simulink model "tpi_sim"  (R2019a)
settings: Solver=VariableStepDiscrete  StartTime=0.0  StopTime=inf  RelTol=1e-3
values from neighbouring files (symbols this model uses):
  tbd1 = 5*(stages1 - 1)    (= 30)    [simloop_and_plot.m]
  tbd2 = 5*(stages2 - 1)    (= 10)    [simloop_and_plot.m]
  tbd3 = 5*(stages3 - 1)    (= 20)    [simloop_and_plot.m]
  tbd4 = 5*(stages4 - 1)    (= 40)    [simloop_and_plot.m]
libraries: commdigbbndpm3 x18, commcnvcod2 x18, commchan3 x14, commutil2 x14, commsink2 x14, commrandsrc3 x14, commdigbbndam3 x8
settings Model: Creator=Lucas  LastModifiedBy=Lucas
settings DataIOCC: LimitDataPoints=on  SaveOutput=off  SaveTime=off
settings OptimizationCC: BooleanDataType=off  DefaultParameterBehavior=Inlined  LocalBlockOutputs=off  LifeSpan=inf
settings DebuggingCC: AlgebraicLoopMsg=error  SingleTaskRateTransMsg=error  AllowSymbolicDim=off  SFUnexpectedBacktrackingDiag=warning  SFNoUnconditionalDefaultTransitionDiag=warning  SFExecutionAtInitializationDiag=none  ArithmeticOperatorsInVariantConditions=warning
settings SFSimCC: SimUseLocalCustomCode=off
settings RTWCC: RTWUseLocalCustomCode=off
settings CodeAppCC: StateflowObjectComments=on
settings GRTTargetCC: TargetLangStandard=C89/C90 (ANSI)  GeneratePreprocessorConditionals=Disable all
settings ConfigComp: CovMetricSettings=dw  CovHtmlReporting=on  CovSaveCumulativeToWorkspaceVar=on  CovSaveSingleToWorkspaceVar=on  CovExternalEMLEnable=off  CovSFcnEnable=off

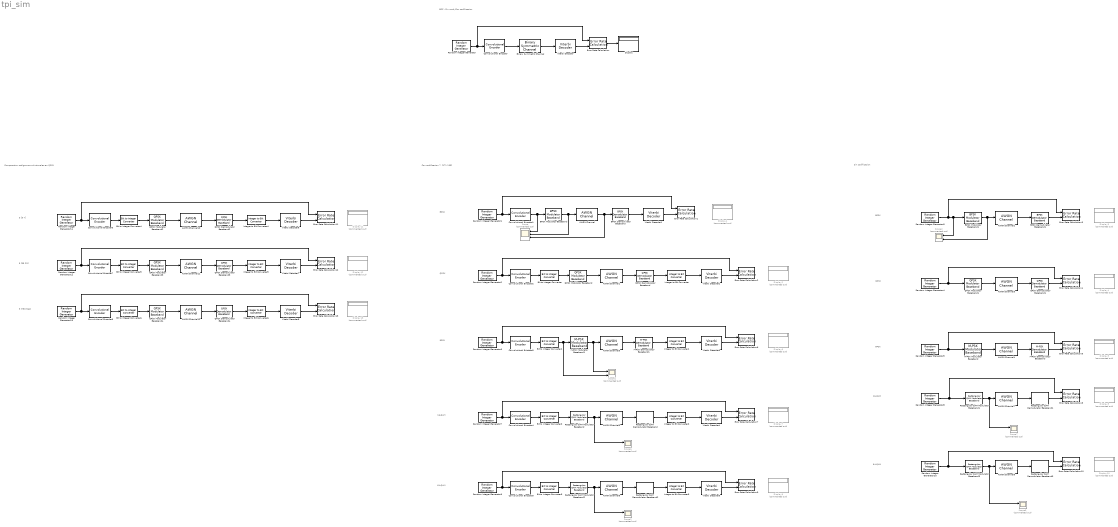
== system tpi_sim ==
  note: BPSK
  note: BSC - Sin mod./Con codificacion
  note: QPSK
  note: 8PSK
  note: 16-QAM
  note: 16-QAM
  note: 64-QAM
  note: 64-QAM
  note: Con codificacion 7, [171 133]
  note: Sin codificacion
  note: 8PSK
  note: QPSK
  note: BPSK
  note: 3 [5 7]
  note: Comparacion codigos convolucionales en QPSK
  note: 5 [35 23]
  note: 9 [753 561]
  AWGN Channel : commchan3/AWGN Channel  InputProcessing=Columns as channels (frame based)  seed=67  noiseMode="Signal to noise ratio  (Eb/No)"  EbNodB=EbNo  EsNodB=10  SNRdB=10  bitsPerSym=1  Ps=1  Tsym=1  variance=1
      settings: SourceProductName=Communications Toolbox
  AWGN Channel{1,10..12} (4 alike) : commchan3/AWGN Channel  InputProcessing=Columns as channels (frame based)  seed=67  noiseMode="Signal to noise ratio  (Eb/No)"  EbNodB=EbNo  EsNodB=10  SNRdB=10  bitsPerSym=2  Ps=1  Tsym=2  variance=1
      settings: SourceProductName=Communications Toolbox
  AWGN Channel2 : commchan3/AWGN Channel  InputProcessing=Columns as channels (frame based)  seed=67  noiseMode="Signal to noise ratio  (Eb/No)"  EbNodB=EbNo  EsNodB=10  SNRdB=10  bitsPerSym=1  Ps=1  Tsym=1  variance=1
      settings: SourceProductName=Communications Toolbox
  AWGN Channel3 : commchan3/AWGN Channel  InputProcessing=Columns as channels (frame based)  seed=67  noiseMode="Signal to noise ratio  (Eb/No)"  EbNodB=EbNo  EsNodB=10  SNRdB=10  bitsPerSym=2  Ps=1  Tsym=1  variance=1
      settings: SourceProductName=Communications Toolbox
  AWGN Channel4 : commchan3/AWGN Channel  InputProcessing=Columns as channels (frame based)  seed=67  noiseMode="Signal to noise ratio  (Eb/No)"  EbNodB=EbNo  EsNodB=10  SNRdB=10  bitsPerSym=3  Ps=1  Tsym=1  variance=1
      settings: SourceProductName=Communications Toolbox
  AWGN Channel5 : commchan3/AWGN Channel  InputProcessing=Columns as channels (frame based)  seed=67  noiseMode="Signal to noise ratio  (Eb/No)"  EbNodB=EbNo  EsNodB=10  SNRdB=10  bitsPerSym=3  Ps=1  Tsym=3  variance=1
      settings: SourceProductName=Communications Toolbox
  AWGN Channel6 : commchan3/AWGN Channel  InputProcessing=Columns as channels (frame based)  seed=67  noiseMode="Signal to noise ratio  (Eb/No)"  EbNodB=EbNo  EsNodB=10  SNRdB=10  bitsPerSym=4  Ps=1  Tsym=2  variance=1
      settings: SourceProductName=Communications Toolbox
  AWGN Channel7 : commchan3/AWGN Channel  InputProcessing=Columns as channels (frame based)  seed=67  noiseMode="Signal to noise ratio  (Eb/No)"  EbNodB=EbNo  EsNodB=10  SNRdB=10  bitsPerSym=4  Ps=1  Tsym=1  variance=1
      settings: SourceProductName=Communications Toolbox
  AWGN Channel8 : commchan3/AWGN Channel  InputProcessing=Columns as channels (frame based)  seed=67  noiseMode="Signal to noise ratio  (Eb/No)"  EbNodB=EbNo  EsNodB=10  SNRdB=10  bitsPerSym=6  Ps=1  Tsym=3  variance=1
      settings: SourceProductName=Communications Toolbox
  AWGN Channel9 : commchan3/AWGN Channel  InputProcessing=Columns as channels (frame based)  seed=67  noiseMode="Signal to noise ratio  (Eb/No)"  EbNodB=EbNo  EsNodB=10  SNRdB=10  bitsPerSym=6  Ps=1  Tsym=1  variance=1
      settings: SourceProductName=Communications Toolbox
  BPSK Demodulator Baseband : commdigbbndpm3/BPSK Demodulator Baseband  DecType=Hard decision  VarSource=Dialog  Variance=1  Ph=0  outDtype=Inherit via internal rule  derotateFactorWordLen=16  derotateFactorDataTypeStr=Inherit: Same word length as input  derotateFactorLastDataTypeStr=Inherit: Same word length as input
      settings: SourceProductName=Communications Toolbox
  BPSK Demodulator Baseband1 : commdigbbndpm3/BPSK Demodulator Baseband  DecType=Hard decision  VarSource=Dialog  Variance=1  Ph=0  outDtype=uint8  derotateFactorWordLen=16  derotateFactorDataTypeStr=Inherit: Same word length as input  derotateFactorLastDataTypeStr=Inherit: Same word length as input
      settings: SourceProductName=Communications Toolbox
  BPSK Modulator Baseband : commdigbbndpm3/BPSK Modulator Baseband  Ph=0  outDtype=double  outWordLen=16  outUDDataType=sfix(16)  outFracLenMode=Best precision  outFracLen=15  outDataTypeStr=double  outLastDataTypeStr=double
      settings: SourceProductName=Communications Toolbox
  BPSK Modulator Baseband1 : commdigbbndpm3/BPSK Modulator Baseband  Ph=0  outDtype=double  outWordLen=16  outUDDataType=sfix(16)  outFracLenMode=Best precision  outFracLen=15  outDataTypeStr=double  outLastDataTypeStr=double
      settings: SourceProductName=Communications Toolbox
  Binary Symmetric Channel : commchan3/Binary Symmetric Channel  ErrorProbability=0.1  ErrorVectorOutputPort=off  OutputDataType=double  OutputDataTypeSL=boolean  Seed=71  SimulateUsing=Code generation
      settings: SourceProductName=Communications Toolbox  SourceProductBaseCode=CM
  Bit to Integer Converter{,4..6} (4 alike) : commutil2/Bit to Integer Converter  nbits=2  bitOrder=MSB first  signedOutputValues=Unsigned  outDtype=Inherit via internal rule  outDtypeSigned=Inherit via internal rule
      settings: SourceProductName=Communications Toolbox
  Bit to Integer Converter1 : commutil2/Bit to Integer Converter  nbits=3  bitOrder=MSB first  signedOutputValues=Unsigned  outDtype=Inherit via internal rule  outDtypeSigned=Inherit via internal rule
      settings: SourceProductName=Communications Toolbox
  Bit to Integer Converter2 : commutil2/Bit to Integer Converter  nbits=4  bitOrder=MSB first  signedOutputValues=Unsigned  outDtype=Inherit via internal rule  outDtypeSigned=Inherit via internal rule
      settings: SourceProductName=Communications Toolbox
  Bit to Integer Converter3 : commutil2/Bit to Integer Converter  nbits=6  bitOrder=MSB first  signedOutputValues=Unsigned  outDtype=Inherit via internal rule  outDtypeSigned=Inherit via internal rule
      settings: SourceProductName=Communications Toolbox
  Convolutional Encoder{,2..5} (5 alike) : commcnvcod2/Convolutional Encoder  trellis=poly2trellis(7, [171 133])  opMode=Continuous  DelayedResetAction=off  hasIniStPort=off  hasFinStPort=off  usePuncVector=off  punctureVector=[1; 1; 0; 1; 0; 1]  reset=Unused parameter value
      settings: SourceProductName=Communications Toolbox  SourceProductBaseCode=CM
  Convolutional Encoder1 : commcnvcod2/Convolutional Encoder  trellis=trellis1  opMode=Continuous  DelayedResetAction=off  hasIniStPort=off  hasFinStPort=off  usePuncVector=off  punctureVector=[1; 1; 0; 1; 0; 1]  reset=Unused parameter value
      settings: SourceProductName=Communications Toolbox  SourceProductBaseCode=CM
  Convolutional Encoder6 : commcnvcod2/Convolutional Encoder  trellis=trellis2  opMode=Continuous  DelayedResetAction=off  hasIniStPort=off  hasFinStPort=off  usePuncVector=off  punctureVector=[1; 1; 0; 1; 0; 1]  reset=Unused parameter value
      settings: SourceProductName=Communications Toolbox  SourceProductBaseCode=CM
  Convolutional Encoder7 : commcnvcod2/Convolutional Encoder  trellis=trellis3  opMode=Continuous  DelayedResetAction=off  hasIniStPort=off  hasFinStPort=off  usePuncVector=off  punctureVector=[1; 1; 0; 1; 0; 1]  reset=Unused parameter value
      settings: SourceProductName=Communications Toolbox  SourceProductBaseCode=CM
  Convolutional Encoder8 : commcnvcod2/Convolutional Encoder  trellis=trellis4  opMode=Continuous  DelayedResetAction=off  hasIniStPort=off  hasFinStPort=off  usePuncVector=off  punctureVector=[1; 1; 0; 1; 0; 1]  reset=Unused parameter value
      settings: SourceProductName=Communications Toolbox  SourceProductBaseCode=CM
  Display : Display
  Display{1..13} (13 alike) : Display  Commented=on
  Error Rate Calculation : commsink2/Error Rate Calculation  N=30  st_delay=0  cp_mode=Entire frame  subframe=[]  PMode=Port  WsName=ErrorVec  RsMode2=off  stop=off  numErr=100  maxBits=1e6
      settings: SourceProductName=Communications Toolbox
  Error Rate Calculation1 : commsink2/Error Rate Calculation  N=tbd1  st_delay=0  cp_mode=Entire frame  subframe=[]  PMode=Workspace  WsName=bpsk_cod  RsMode2=off  stop=on  numErr=inf  maxBits=max_symbols
      settings: SourceProductName=Communications Toolbox
  Error Rate Calculation10 : commsink2/Error Rate Calculation  N=0  st_delay=0  cp_mode=Entire frame  subframe=[1;0;0]  PMode=Workspace  WsName=qam64  RsMode2=off  stop=off  numErr=100  maxBits=1e6
      settings: SourceProductName=Communications Toolbox
  Error Rate Calculation11 : commsink2/Error Rate Calculation  N=tbd2  st_delay=0  cp_mode=Entire frame  subframe=[]  PMode=Workspace  WsName=cod2  RsMode2=off  stop=off  numErr=inf  maxBits=1e4
      settings: SourceProductName=Communications Toolbox
  Error Rate Calculation12 : commsink2/Error Rate Calculation  N=tbd3  st_delay=0  cp_mode=Entire frame  subframe=[]  PMode=Workspace  WsName=cod3  RsMode2=off  stop=off  numErr=inf  maxBits=1e4
      settings: SourceProductName=Communications Toolbox
  Error Rate Calculation13 : commsink2/Error Rate Calculation  N=tbd4  st_delay=0  cp_mode=Entire frame  subframe=[]  PMode=Workspace  WsName=cod4  RsMode2=off  stop=off  numErr=inf  maxBits=1e4
      settings: SourceProductName=Communications Toolbox
  Error Rate Calculation2 : commsink2/Error Rate Calculation  N=tbd1  st_delay=0  cp_mode=Entire frame  subframe=[]  PMode=Workspace  WsName=qpsk_cod  RsMode2=off  stop=off  numErr=inf  maxBits=1e4
      settings: SourceProductName=Communications Toolbox
  Error Rate Calculation3 : commsink2/Error Rate Calculation  N=0  st_delay=0  cp_mode=Entire frame  subframe=[]  PMode=Workspace  WsName=bpsk  RsMode2=off  stop=off  numErr=100  maxBits=1e6
      settings: SourceProductName=Communications Toolbox
  Error Rate Calculation4 : commsink2/Error Rate Calculation  N=0  st_delay=0  cp_mode=Entire frame  subframe=[]  PMode=Workspace  WsName=qpsk  RsMode2=off  stop=off  numErr=100  maxBits=1e6
      settings: SourceProductName=Communications Toolbox
  Error Rate Calculation5 : commsink2/Error Rate Calculation  N=0  st_delay=0  cp_mode=Entire frame  subframe=[]  PMode=Workspace  WsName=psk8  RsMode2=off  stop=off  numErr=100  maxBits=1e6
      settings: SourceProductName=Communications Toolbox
  Error Rate Calculation6 : commsink2/Error Rate Calculation  N=tbd1  st_delay=0  cp_mode=Entire frame  subframe=[1;0;0]  PMode=Workspace  WsName=psk8_cod  RsMode2=off  stop=off  numErr=100  maxBits=1e6
      settings: SourceProductName=Communications Toolbox
  Error Rate Calculation7 : commsink2/Error Rate Calculation  N=tbd1  st_delay=0  cp_mode=Entire frame  subframe=[1;0;0]  PMode=Workspace  WsName=qam16_cod  RsMode2=off  stop=off  numErr=100  maxBits=1e6
      settings: SourceProductName=Communications Toolbox
  Error Rate Calculation8 : commsink2/Error Rate Calculation  N=0  st_delay=0  cp_mode=Entire frame  subframe=[1;0;0]  PMode=Workspace  WsName=qam16  RsMode2=off  stop=off  numErr=100  maxBits=1e6
      settings: SourceProductName=Communications Toolbox
  Error Rate Calculation9 : commsink2/Error Rate Calculation  N=tbd1  st_delay=0  cp_mode=Entire frame  subframe=[1;0;0]  PMode=Workspace  WsName=qam64_cod  RsMode2=off  stop=off  numErr=100  maxBits=1e6
      settings: SourceProductName=Communications Toolbox
  Integer to Bit Converter{,4..6} (4 alike) : commutil2/Integer to Bit Converter  nbits=2  signedInputValues=Unsigned  bitOrder=MSB first  outDtype=Inherit via internal rule
      settings: SourceProductName=Communications Toolbox
  Integer to Bit Converter1 : commutil2/Integer to Bit Converter  nbits=3  signedInputValues=Unsigned  bitOrder=MSB first  outDtype=Inherit via internal rule
      settings: SourceProductName=Communications Toolbox
  Integer to Bit Converter2 : commutil2/Integer to Bit Converter  nbits=4  signedInputValues=Unsigned  bitOrder=MSB first  outDtype=Inherit via internal rule
      settings: SourceProductName=Communications Toolbox
  Integer to Bit Converter3 : commutil2/Integer to Bit Converter  nbits=6  signedInputValues=Unsigned  bitOrder=MSB first  outDtype=Inherit via internal rule
      settings: SourceProductName=Communications Toolbox
  M-PSK Demodulator Baseband : commdigbbndpm3/M-PSK Demodulator Baseband  M=8  OutType=Integer  DecType=Hard decision  VarSource=Dialog  Variance=1  Dec=Gray  Mapping=[0:7]  Ph=pi/8  outDtype1=Inherit via internal rule  outDtype2=Inherit via internal rule  derotateFactorWordLen=16  derotateFactorDataTypeStr=Inherit: Same word length as input  derotateFactorLastDataTypeStr=Inherit: Same word length as input
      settings: SourceProductName=Communications Toolbox
  M-PSK Demodulator Baseband1 : commdigbbndpm3/M-PSK Demodulator Baseband  M=8  OutType=Integer  DecType=Hard decision  VarSource=Dialog  Variance=1  Dec=Gray  Mapping=[0:7]  Ph=pi/8  outDtype1=Inherit via internal rule  outDtype2=uint8  derotateFactorWordLen=16  derotateFactorDataTypeStr=Inherit: Same word length as input  derotateFactorLastDataTypeStr=Inherit: Same word length as input
      settings: SourceProductName=Communications Toolbox
  M-PSK Modulator Baseband : commdigbbndpm3/M-PSK Modulator Baseband  M=8  InType=Integer  Enc=Gray  Mapping=[0:7]  Ph=pi/8  outDtype=double  outWordLen=16  outUDDataType=sfix(16)  outFracLenMode=Best precision  outFracLen=15  outDataTypeStr=double  outLastDataTypeStr=double
      settings: SourceProductName=Communications Toolbox
  M-PSK Modulator Baseband1 : commdigbbndpm3/M-PSK Modulator Baseband  M=8  InType=Integer  Enc=Gray  Mapping=[0:7]  Ph=pi/8  outDtype=double  outWordLen=16  outUDDataType=sfix(16)  outFracLenMode=Best precision  outFracLen=15  outDataTypeStr=double  outLastDataTypeStr=double
      settings: SourceProductName=Communications Toolbox
  QPSK Demodulator Baseband{,1..4} (5 alike) : commdigbbndpm3/QPSK Demodulator Baseband  OutType=Integer  DecType=Hard decision  VarSource=Dialog  Variance=1  Dec=Gray  Ph=pi/4  outDtype1=Inherit via internal rule  outDtype2=uint8  derotateFactorWordLen=16  derotateFactorDataTypeStr=Inherit: Same word length as input  derotateFactorLastDataTypeStr=Inherit: Same word length as input
      settings: SourceProductName=Communications Toolbox
  QPSK Modulator Baseband{,1..4} (5 alike) : commdigbbndpm3/QPSK Modulator Baseband  InType=Integer  Enc=Gray  Ph=pi/4  outDtype=double  outWordLen=16  outUDDataType=sfix(16)  outFracLenMode=Best precision  outFracLen=15  outDataTypeStr=double  outLastDataTypeStr=double
      settings: SourceProductName=Communications Toolbox
  Random Integer Generator : commrandsrc3/Random Integer Generator  SetSize=2  SeedSource=Auto  Seed=0  SampleTime=1  SamplesPerFrame=1  OutputDataType=boolean  SimulateUsing=Code generation
      settings: SourceProductName=Communications Toolbox
  Random Integer Generator1 : commrandsrc3/Random Integer Generator  SetSize=2  SeedSource=Auto  Seed=0  SampleTime=1  SamplesPerFrame=1  OutputDataType=boolean  SimulateUsing=Code generation
      settings: SourceProductName=Communications Toolbox
  Random Integer Generator10 : commrandsrc3/Random Integer Generator  SetSize=6  SeedSource=Auto  Seed=0  SampleTime=1  SamplesPerFrame=1  OutputDataType=uint8  SimulateUsing=Code generation
      settings: SourceProductName=Communications Toolbox
  Random Integer Generator{2,7,11..13} (5 alike) : commrandsrc3/Random Integer Generator  SetSize=2  SeedSource=Auto  Seed=0  SampleTime=1  SamplesPerFrame=2  OutputDataType=uint8  SimulateUsing=Code generation
      settings: SourceProductName=Communications Toolbox
  Random Integer Generator3 : commrandsrc3/Random Integer Generator  SetSize=2  SeedSource=Auto  Seed=0  SampleTime=1  SamplesPerFrame=1  OutputDataType=uint8  SimulateUsing=Code generation
      settings: SourceProductName=Communications Toolbox
  Random Integer Generator4 : commrandsrc3/Random Integer Generator  SetSize=4  SeedSource=Auto  Seed=5  SampleTime=1  SamplesPerFrame=1  OutputDataType=uint8  SimulateUsing=Code generation
      settings: SourceProductName=Communications Toolbox
  Random Integer Generator5 : commrandsrc3/Random Integer Generator  SetSize=8  SeedSource=Auto  Seed=5  SampleTime=1  SamplesPerFrame=1  OutputDataType=uint8  SimulateUsing=Code generation
      settings: SourceProductName=Communications Toolbox
  Random Integer Generator6 : commrandsrc3/Random Integer Generator  SetSize=2  SeedSource=Auto  Seed=0  SampleTime=1  SamplesPerFrame=3  OutputDataType=uint8  SimulateUsing=Code generation
      settings: SourceProductName=Communications Toolbox
  Random Integer Generator8 : commrandsrc3/Random Integer Generator  SetSize=4  SeedSource=Auto  Seed=0  SampleTime=1  SamplesPerFrame=1  OutputDataType=uint8  SimulateUsing=Code generation
      settings: SourceProductName=Communications Toolbox
  Random Integer Generator9 : commrandsrc3/Random Integer Generator  SetSize=2  SeedSource=Auto  Seed=0  SampleTime=1  SamplesPerFrame=3  OutputDataType=uint8  SimulateUsing=Code generation
      settings: SourceProductName=Communications Toolbox
  Rectangular QAM Demodulator Baseband : commdigbbndam3/Rectangular QAM Demodulator Baseband  M=16  OutType=Integer  DecType=Hard decision  VarSource=Dialog  Variance=1  Dec=Gray  Mapping=[0:15]  PowType=Average Power  MinDist=2  AvgPow=1  PeakPow=1  Ph=0  outDtype1=Inherit via internal rule  outDtype2=Inherit via internal rule  derotateFactorWordLen=16  derotateFactorDataTypeStr=Inherit: Same word length as input  derotateFactorLastDataTypeStr=Inherit: Same word length as input  denormFactorWordLen=16  denormFactorDataTypeStr=Inherit: Same word length as input  denormFactorLastDataTypeStr=Inherit: Same word length as input  prodOutWordLen=32  prodOutOverflowMode=Wrap  prodOutRoundingMode=Floor  prodOutOvFlMode=off  prodOutOvFlModeLastStrValue=off  sumWordLen=32
      settings: SourceProductName=Communications Toolbox
  Rectangular QAM Demodulator Baseband1 : commdigbbndam3/Rectangular QAM Demodulator Baseband  M=16  OutType=Integer  DecType=Hard decision  VarSource=Dialog  Variance=1  Dec=Gray  Mapping=[0:15]  PowType=Average Power  MinDist=2  AvgPow=1  PeakPow=1  Ph=0  outDtype1=Inherit via internal rule  outDtype2=Inherit via internal rule  derotateFactorWordLen=16  derotateFactorDataTypeStr=Inherit: Same word length as input  derotateFactorLastDataTypeStr=Inherit: Same word length as input  denormFactorWordLen=16  denormFactorDataTypeStr=Inherit: Same word length as input  denormFactorLastDataTypeStr=Inherit: Same word length as input  prodOutWordLen=32  prodOutOverflowMode=Wrap  prodOutRoundingMode=Floor  prodOutOvFlMode=off  prodOutOvFlModeLastStrValue=off  sumWordLen=32
      settings: SourceProductName=Communications Toolbox
  Rectangular QAM Demodulator Baseband2 : commdigbbndam3/Rectangular QAM Demodulator Baseband  M=64  OutType=Integer  DecType=Hard decision  VarSource=Dialog  Variance=1  Dec=Gray  Mapping=[0:15]  PowType=Average Power  MinDist=2  AvgPow=1  PeakPow=1  Ph=0  outDtype1=Inherit via internal rule  outDtype2=Inherit via internal rule  derotateFactorWordLen=16  derotateFactorDataTypeStr=Inherit: Same word length as input  derotateFactorLastDataTypeStr=Inherit: Same word length as input  denormFactorWordLen=16  denormFactorDataTypeStr=Inherit: Same word length as input  denormFactorLastDataTypeStr=Inherit: Same word length as input  prodOutWordLen=32  prodOutOverflowMode=Wrap  prodOutRoundingMode=Floor  prodOutOvFlMode=off  prodOutOvFlModeLastStrValue=off  sumWordLen=32
      settings: SourceProductName=Communications Toolbox
  Rectangular QAM Demodulator Baseband3 : commdigbbndam3/Rectangular QAM Demodulator Baseband  M=64  OutType=Integer  DecType=Hard decision  VarSource=Dialog  Variance=1  Dec=Gray  Mapping=[0:15]  PowType=Average Power  MinDist=2  AvgPow=1  PeakPow=1  Ph=0  outDtype1=Inherit via internal rule  outDtype2=Inherit via internal rule  derotateFactorWordLen=16  derotateFactorDataTypeStr=Inherit: Same word length as input  derotateFactorLastDataTypeStr=Inherit: Same word length as input  denormFactorWordLen=16  denormFactorDataTypeStr=Inherit: Same word length as input  denormFactorLastDataTypeStr=Inherit: Same word length as input  prodOutWordLen=32  prodOutOverflowMode=Wrap  prodOutRoundingMode=Floor  prodOutOvFlMode=off  prodOutOvFlModeLastStrValue=off  sumWordLen=32
      settings: SourceProductName=Communications Toolbox
  Rectangular QAM Modulator Baseband : commdigbbndam3/Rectangular QAM Modulator Baseband  M=16  InType=Integer  Enc=Gray  Mapping=[0:15]  PowType=Average Power  MinDist=2  AvgPow=1  PeakPow=1  Ph=0  outDtype=double  outWordLen=16  outUDDataType=sfix(16)  outFracLenMode=Best precision  outFracLen=15  outDataTypeStr=double  outLastDataTypeStr=double
      settings: SourceProductName=Communications Toolbox
  Rectangular QAM Modulator Baseband1 : commdigbbndam3/Rectangular QAM Modulator Baseband  M=16  InType=Integer  Enc=Gray  Mapping=[0:15]  PowType=Average Power  MinDist=2  AvgPow=1  PeakPow=1  Ph=0  outDtype=double  outWordLen=16  outUDDataType=sfix(16)  outFracLenMode=Best precision  outFracLen=15  outDataTypeStr=double  outLastDataTypeStr=double
      settings: SourceProductName=Communications Toolbox
  Rectangular QAM Modulator Baseband2 : commdigbbndam3/Rectangular QAM Modulator Baseband  M=64  InType=Integer  Enc=Gray  Mapping=[0:15]  PowType=Average Power  MinDist=2  AvgPow=1  PeakPow=1  Ph=0  outDtype=double  outWordLen=16  outUDDataType=sfix(16)  outFracLenMode=Best precision  outFracLen=15  outDataTypeStr=double  outLastDataTypeStr=double
      settings: SourceProductName=Communications Toolbox
  Rectangular QAM Modulator Baseband3 : commdigbbndam3/Rectangular QAM Modulator Baseband  M=64  InType=Integer  Enc=Gray  Mapping=[0:15]  PowType=Average Power  MinDist=2  AvgPow=1  PeakPow=1  Ph=0  outDtype=double  outWordLen=16  outUDDataType=sfix(16)  outFracLenMode=Best precision  outFracLen=15  outDataTypeStr=double  outLastDataTypeStr=double
      settings: SourceProductName=Communications Toolbox
  Scope : Scope  Commented=on  NumInputPorts=3
  Scope{1..3,6..7,9} (6 alike) : Scope  Commented=on  NumInputPorts=2
  Viterbi Decoder : commcnvcod2/Viterbi Decoder  trellis=poly2trellis(7, [171 133])  isPunctured=off  punctureVector=[1; 1; 0; 1; 0; 1]  erasures=off  dectype=Hard decision  nsdecb=4  runSigValErrCheck=off  tbdepth=30  opmode=Continuous  reset=off  delayedResetAction=off  smWordLength=16  outDataType=boolean
      settings: SourceProductName=Communications Toolbox  SourceProductBaseCode=CM
  Viterbi Decoder1 : commcnvcod2/Viterbi Decoder  trellis=trellis1  isPunctured=off  punctureVector=[1; 1; 0; 1; 0; 1]  erasures=off  dectype=Hard decision  nsdecb=4  runSigValErrCheck=off  tbdepth=tbd1  opmode=Continuous  reset=off  delayedResetAction=off  smWordLength=16  outDataType=boolean
      settings: SourceProductName=Communications Toolbox  SourceProductBaseCode=CM
  Viterbi Decoder{2..5} (4 alike) : commcnvcod2/Viterbi Decoder  trellis=poly2trellis(7, [171 133])  isPunctured=off  punctureVector=[1; 1; 0; 1; 0; 1]  erasures=off  dectype=Hard decision  nsdecb=4  runSigValErrCheck=off  tbdepth=30  opmode=Continuous  reset=off  delayedResetAction=off  smWordLength=16  outDataType=uint8
      settings: SourceProductName=Communications Toolbox  SourceProductBaseCode=CM
  Viterbi Decoder6 : commcnvcod2/Viterbi Decoder  trellis=trellis2  isPunctured=off  punctureVector=[1; 1; 0; 1; 0; 1]  erasures=off  dectype=Hard decision  nsdecb=4  runSigValErrCheck=off  tbdepth=tbd2  opmode=Continuous  reset=off  delayedResetAction=off  smWordLength=16  outDataType=uint8
      settings: SourceProductName=Communications Toolbox  SourceProductBaseCode=CM
  Viterbi Decoder7 : commcnvcod2/Viterbi Decoder  trellis=trellis3  isPunctured=off  punctureVector=[1; 1; 0; 1; 0; 1]  erasures=off  dectype=Hard decision  nsdecb=4  runSigValErrCheck=off  tbdepth=tbd3  opmode=Continuous  reset=off  delayedResetAction=off  smWordLength=16  outDataType=uint8
      settings: SourceProductName=Communications Toolbox  SourceProductBaseCode=CM
  Viterbi Decoder8 : commcnvcod2/Viterbi Decoder  trellis=trellis4  isPunctured=off  punctureVector=[1; 1; 0; 1; 0; 1]  erasures=off  dectype=Hard decision  nsdecb=4  runSigValErrCheck=off  tbdepth=tbd4  opmode=Continuous  reset=off  delayedResetAction=off  smWordLength=16  outDataType=uint8
      settings: SourceProductName=Communications Toolbox  SourceProductBaseCode=CM
  wires:
  Random Integer Generator/1 -> Error Rate Calculation/1, Convolutional Encoder/1
  Convolutional Encoder/1 -> Binary Symmetric Channel/1
  Viterbi Decoder/1 -> Error Rate Calculation/2
  Error Rate Calculation/1 -> Display/1
  Binary Symmetric Channel/1 -> Viterbi Decoder/1
  Viterbi Decoder1/1 -> Error Rate Calculation1/2
  Random Integer Generator1/1 -> Error Rate Calculation1/1, Convolutional Encoder1/1
  Convolutional Encoder1/1 -> Scope/1, BPSK Modulator Baseband/1
  BPSK Modulator Baseband/1 -> Scope/2, AWGN Channel/1
  AWGN Channel/1 -> Scope/3, BPSK Demodulator Baseband/1
  BPSK Demodulator Baseband/1 -> Viterbi Decoder1/1
  AWGN Channel1/1 -> QPSK Demodulator Baseband/1
  QPSK Modulator Baseband/1 -> AWGN Channel1/1
  Convolutional Encoder2/1 -> Bit to Integer Converter/1
  Random Integer Generator2/1 -> Convolutional Encoder2/1, Error Rate Calculation2/1
  Viterbi Decoder2/1 -> Error Rate Calculation2/2
  Bit to Integer Converter/1 -> QPSK Modulator Baseband/1
  QPSK Demodulator Baseband/1 -> Integer to Bit Converter/1
  Integer to Bit Converter/1 -> Viterbi Decoder2/1
  QPSK Modulator Baseband1/1 -> AWGN Channel3/1
  AWGN Channel3/1 -> QPSK Demodulator Baseband1/1
  AWGN Channel2/1 -> BPSK Demodulator Baseband1/1
  BPSK Modulator Baseband1/1 -> Scope2/2, AWGN Channel2/1
  Random Integer Generator3/1 -> Scope2/1, BPSK Modulator Baseband1/1, Error Rate Calculation3/1
  BPSK Demodulator Baseband1/1 -> Error Rate Calculation3/2
  Random Integer Generator4/1 -> QPSK Modulator Baseband1/1, Error Rate Calculation4/1
  QPSK Demodulator Baseband1/1 -> Error Rate Calculation4/2
  M-PSK Demodulator Baseband/1 -> Error Rate Calculation5/2
  Random Integer Generator5/1 -> M-PSK Modulator Baseband/1, Error Rate Calculation5/1
  AWGN Channel4/1 -> M-PSK Demodulator Baseband/1
  M-PSK Modulator Baseband/1 -> AWGN Channel4/1
  Integer to Bit Converter1/1 -> Viterbi Decoder3/1
  M-PSK Demodulator Baseband1/1 -> Integer to Bit Converter1/1
  Bit to Integer Converter1/1 -> Scope1/2, M-PSK Modulator Baseband1/1
  Viterbi Decoder3/1 -> Error Rate Calculation6/2
  Random Integer Generator6/1 -> Error Rate Calculation6/1, Convolutional Encoder3/1
  Convolutional Encoder3/1 -> Bit to Integer Converter1/1
  M-PSK Modulator Baseband1/1 -> Scope1/1, AWGN Channel5/1
  AWGN Channel5/1 -> M-PSK Demodulator Baseband1/1
  Convolutional Encoder4/1 -> Bit to Integer Converter2/1
  Random Integer Generator7/1 -> Convolutional Encoder4/1, Error Rate Calculation7/1
  Viterbi Decoder4/1 -> Error Rate Calculation7/2
  Integer to Bit Converter2/1 -> Viterbi Decoder4/1
  Rectangular QAM Demodulator Baseband/1 -> Integer to Bit Converter2/1
  AWGN Channel6/1 -> Rectangular QAM Demodulator Baseband/1
  Rectangular QAM Modulator Baseband/1 -> Scope6/1, AWGN Channel6/1
  Bit to Integer Converter2/1 -> Rectangular QAM Modulator Baseband/1
  Random Integer Generator8/1 -> Rectangular QAM Modulator Baseband1/1, Error Rate Calculation8/1
  Rectangular QAM Modulator Baseband1/1 -> AWGN Channel7/1, Scope7/1
  AWGN Channel7/1 -> Rectangular QAM Demodulator Baseband1/1
  Rectangular QAM Demodulator Baseband1/1 -> Error Rate Calculation8/2
  Rectangular QAM Demodulator Baseband3/1 -> Error Rate Calculation10/2
  AWGN Channel9/1 -> Rectangular QAM Demodulator Baseband3/1
  Rectangular QAM Modulator Baseband3/1 -> Scope9/1, AWGN Channel9/1
  Random Integer Generator10/1 -> Error Rate Calculation10/1, Rectangular QAM Modulator Baseband3/1
  Bit to Integer Converter3/1 -> Rectangular QAM Modulator Baseband2/1
  Rectangular QAM Modulator Baseband2/1 -> AWGN Channel8/1, Scope3/1
  AWGN Channel8/1 -> Rectangular QAM Demodulator Baseband2/1
  Rectangular QAM Demodulator Baseband2/1 -> Integer to Bit Converter3/1
  Integer to Bit Converter3/1 -> Viterbi Decoder5/1
  Viterbi Decoder5/1 -> Error Rate Calculation9/2
  Random Integer Generator9/1 -> Error Rate Calculation9/1, Convolutional Encoder5/1
  Convolutional Encoder5/1 -> Bit to Integer Converter3/1
  Integer to Bit Converter4/1 -> Viterbi Decoder6/1
  QPSK Demodulator Baseband2/1 -> Integer to Bit Converter4/1
  Bit to Integer Converter4/1 -> QPSK Modulator Baseband2/1
  Viterbi Decoder6/1 -> Error Rate Calculation11/2
  Random Integer Generator11/1 -> Error Rate Calculation11/1, Convolutional Encoder6/1
  Convolutional Encoder6/1 -> Bit to Integer Converter4/1
  QPSK Modulator Baseband2/1 -> AWGN Channel10/1
  AWGN Channel10/1 -> QPSK Demodulator Baseband2/1
  AWGN Channel11/1 -> QPSK Demodulator Baseband3/1
  QPSK Modulator Baseband3/1 -> AWGN Channel11/1
  Convolutional Encoder7/1 -> Bit to Integer Converter5/1
  Random Integer Generator12/1 -> Convolutional Encoder7/1, Error Rate Calculation12/1
  Viterbi Decoder7/1 -> Error Rate Calculation12/2
  Bit to Integer Converter5/1 -> QPSK Modulator Baseband3/1
  QPSK Demodulator Baseband3/1 -> Integer to Bit Converter5/1
  Integer to Bit Converter5/1 -> Viterbi Decoder7/1
  Integer to Bit Converter6/1 -> Viterbi Decoder8/1
  QPSK Demodulator Baseband4/1 -> Integer to Bit Converter6/1
  Bit to Integer Converter6/1 -> QPSK Modulator Baseband4/1
  Viterbi Decoder8/1 -> Error Rate Calculation13/2
  Random Integer Generator13/1 -> Error Rate Calculation13/1, Convolutional Encoder8/1
  Convolutional Encoder8/1 -> Bit to Integer Converter6/1
  QPSK Modulator Baseband4/1 -> AWGN Channel12/1
  AWGN Channel12/1 -> QPSK Demodulator Baseband4/1
